simulink model "Cascade_Realization"  (R2020a)
settings: Solver=VariableStepAuto  StartTime=0.0  StopTime=10.0  RelTol=1e-3
settings Model: Creator=tanu  LastModifiedBy=tanu
settings DataIOCC: SaveOutput=off  SaveTime=off

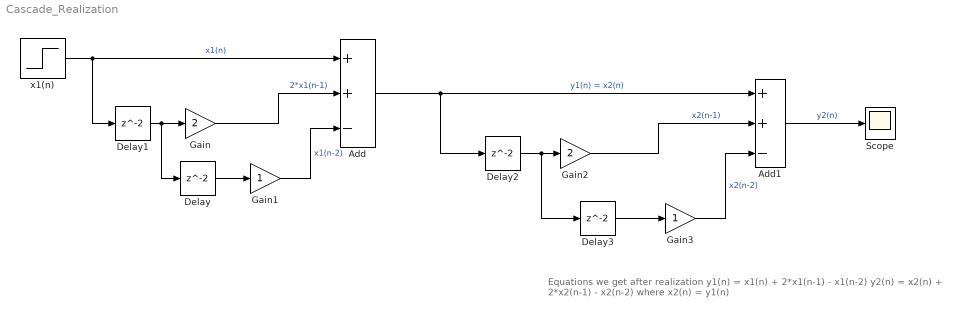
== system Cascade_Realization ==
  note: Equations we get after realization
      | y1(n) = x1(n) + 2*x1(n-1) - x1(n-2)
      | y2(n) = x2(n) + 2*x2(n-1) - x2(n-2)
      |
      | where x2(n) = y1(n)
  Add : Sum  Inputs=++-
  Add1 : Sum  Inputs=++-
  Delay{,1..3} (4 alike) : Delay
  Gain : Gain  Gain=2
  Gain1 : Gain
  Gain2 : Gain  Gain=2
  Gain3 : Gain
  Scope : Scope
  x1(n) : Step  SampleTime=0
  wires:
  Delay1/1 -> Gain/1, Delay/1
  Delay2/1 -> Gain2/1, Delay3/1
  x1(n)/1 -> Add/1, Delay1/1  "x1(n)"
  Gain2/1 -> Add1/2  "x2(n-1)"
  Gain/1 -> Add/2  "2*x1(n-1)"
  Gain1/1 -> Add/3  "x1(n-2)"
  Add/1 -> Delay2/1, Add1/1  "y1(n) = x2(n)"
  Delay/1 -> Gain1/1
  Add1/1 -> Scope/1  "y2(n)"
  Delay3/1 -> Gain3/1
  Gain3/1 -> Add1/3  "x2(n-2)"
